simulink model "project"  (R2019b)
settings: Solver=VariableStepAuto  StartTime=0.0  StopTime=10.0  RelTol=1e-3
values from neighbouring files (symbols this model uses):
  s = profile.o_signals(1,:)    [project_main.m]
settings Model: Creator=markwilkinson  LastModifiedBy=markwilkinson

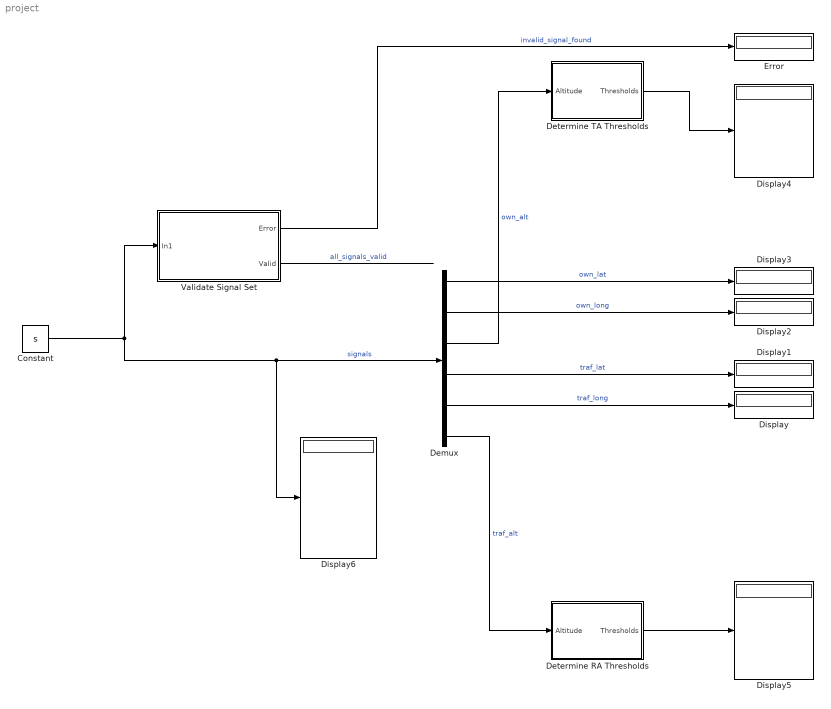
== system project ==
  Constant : Constant  Value=s
  Demux : Demux  Outputs=6
  Determine RA Thresholds : Subsystem
  Determine TA Thresholds : Subsystem
  Display{,1..6} (7 alike) : Display
  "Error " : Display
  "Validate Signal Set " : Subsystem
  wires:
  "Validate Signal Set "/1(Error) -> "Error "/1  "invalid_signal_found"
  "Validate Signal Set "/2(Valid) -> ?  "all_signals_valid"
  Constant/1 -> Display6/1, Demux/1, "Validate Signal Set "/1(In1)  "signals"
  Demux/3 -> Determine TA Thresholds/1(Altitude)  "own_alt"
  Demux/6 -> Determine RA Thresholds/1(Altitude)  "traf_alt"
  Demux/5 -> Display/1  "traf_long"
  Demux/4 -> Display1/1  "traf_lat"
  Demux/2 -> Display2/1  "own_long"
  Demux/1 -> Display3/1  "own_lat"
  Determine TA Thresholds/1(Thresholds) -> Display4/1
  Determine RA Thresholds/1(Thresholds) -> Display5/1

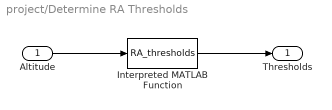
== system project/Determine RA Thresholds ==
  Altitude : Inport
  Interpreted MATLAB Function : MATLABFcn  MATLABFcn=RA_thresholds
  Thresholds : Outport
  wires:
  Altitude/1 -> Interpreted MATLAB Function/1
  Interpreted MATLAB Function/1 -> Thresholds/1

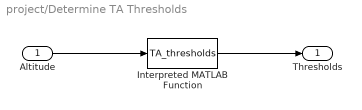
== system project/Determine TA Thresholds ==
  Altitude : Inport
  Interpreted MATLAB Function : MATLABFcn  MATLABFcn=TA_thresholds
  Thresholds : Outport
  wires:
  Altitude/1 -> Interpreted MATLAB Function/1
  Interpreted MATLAB Function/1 -> Thresholds/1

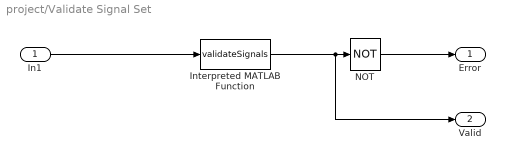
== system project/Validate Signal Set  ==
  In1 : Inport
  Interpreted MATLAB Function : MATLABFcn  MATLABFcn=validateSignals
  NOT : Logic  Operator=NOT  IconShape=distinctive  AllPortsSameDT=off  OutDataTypeStr=boolean
  Error : Outport
  Valid : Outport  Port=2
  wires:
  In1/1 -> Interpreted MATLAB Function/1
  Interpreted MATLAB Function/1 -> Valid/1, NOT/1
  NOT/1 -> Error/1
